simulink model "DoorSystem_Test"  (R2019b)
settings: Solver=ode1  StartTime=0.0  StopTime=inf  FixedStep=0.05  RelTol=1e-3  EnableMultiTasking=on
PostLoadFcn:
  | set_up_test_model
undefined symbols (not defined in the file): Enabled, MaxVehicles, Orientation, Z_DoorSystemPrm
libraries: TestBenchLib x22
settings Model: EnablePacing=on  OrderedModelArguments=off  Creator=godoyb  LastModifiedBy=bnadpurohit
settings DataIOCC: LimitDataPoints=on  ReturnWorkspaceOutputs=off
settings OptimizationCC: DefaultParameterBehavior=Inlined  LifeSpan=inf
settings DebuggingCC: FrameProcessingCompatibilityMsg=warning  AllowSymbolicDim=off  SFUnexpectedBacktrackingDiag=warning  SFNoUnconditionalDefaultTransitionDiag=warning  SFExecutionAtInitializationDiag=none  ArithmeticOperatorsInVariantConditions=warning
settings HardwareCC: ProdBitPerPointer=32  ProdBitPerSizeT=32  ProdBitPerPtrDiffT=32  ProdLargestAtomicFloat=None  ProdIntDivRoundTo=Undefined  ProdEndianess=Unspecified  ProdWordSize=32  ProdHWDeviceType=Custom Processor->Custom
settings ModelReferenceCC: PropagateSignalLabelsOutOfModel=off
settings SFSimCC: SimUseLocalCustomCode=off  CustomCodeUndefinedFunction=UseInterfaceOnly
settings RTWCC: RTWUseLocalCustomCode=off  TargetLang=C++
settings CodeAppCC: StateflowObjectComments=on
settings GRTTargetCC: TargetLangStandard=C++03 (ISO)  MultiInstanceERTCode=on  CodeInterfacePackaging=C++ class
settings ConfigComp: CovMetricSettings=dw  CovHtmlReporting=on  CovSaveCumulativeToWorkspaceVar=on  CovSaveSingleToWorkspaceVar=on  CovExternalEMLEnable=off

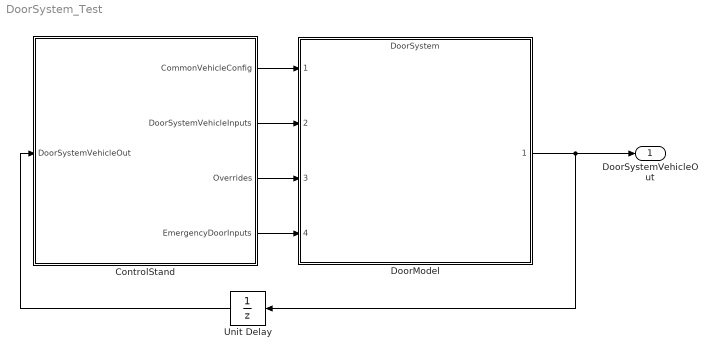
== system DoorSystem_Test ==
  ControlStand : Subsystem
  DoorModel : ModelReference  ModelNameDialog=DoorSystem.slx  ParameterArgumentNames=PRM_DoorSystem  ParameterArgumentValues=[Z_DoorSystemPrm]  UsingDefaultArgumentValue=0  SimulationMode=Normal  ModelReferenceVersion=1.2191
  Unit Delay : UnitDelay  SampleTime=-1  HasFrameUpgradeWarning=on
  DoorSystemVehicleOut : Outport  VectorParamsAs1DForOutWhenUnconnected=off
  wires:
  DoorModel/1 -> Unit Delay/1, DoorSystemVehicleOut/1
  ControlStand/1(CommonVehicleConfig) -> DoorModel/1
  ControlStand/2(DoorSystemVehicleInputs) -> DoorModel/2
  ControlStand/3(Overrides) -> DoorModel/3
  Unit Delay/1 -> ControlStand/1(DoorSystemVehicleOut)
  ControlStand/4(EmergencyDoorInputs) -> DoorModel/4

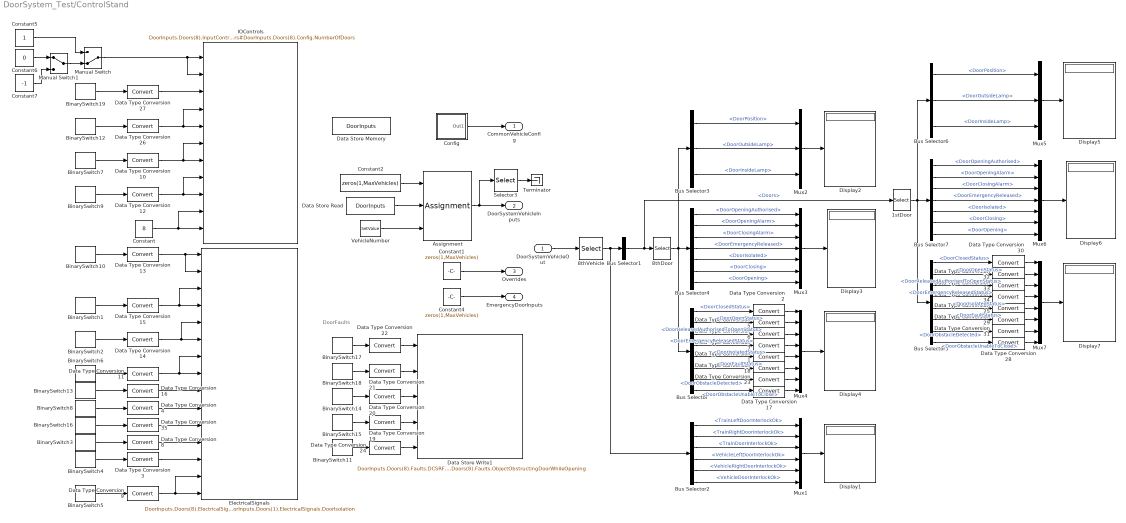
== system DoorSystem_Test/ControlStand ==
  note: DoorFaults
  DoorSystemVehicleOut : Inport
  1stDoor : Selector  InputPortWidth=16  IndexOptions=Index vector (dialog)  Indices=1  OutputSizes=1
  8thDoor : Selector  InputPortWidth=16  IndexOptions=Index vector (dialog)  Indices=16  OutputSizes=1
  8thVehicle : Selector  InputPortWidth=MaxVehicles  IndexOptions=Index vector (dialog)  Indices=8  OutputSizes=1
  Assignment : Assignment  DiagnosticForDimensions=Warning  IndexOptions=Index vector (port)  Indices=1  OutputSizes=1
  BinarySwitch{1..2,6,10} (4 alike) : TestBenchLib/BinarySwitch  value=1  init_value=1  block_colour=[0 1 0]  WorkspaceVarName=0
      settings: SourceProductName=Sydac Utilities
  BinarySwitch{3..5,7..9,11..19} (15 alike) : TestBenchLib/BinarySwitch  value=0  init_value=0  block_colour=[0 1 0]  WorkspaceVarName=0
      settings: SourceProductName=Sydac Utilities
  Bus Selector : BusSelector  OutputSignals=TCMS.DoorClosedStatus,TCMS.DoorOpenStatus,TCMS.DoorReleasedAuthorisedToOpenStatus,TCMS.DoorEmergencyReleasedStatus,TCMS.DoorIsolatedStatus,TCMS.DoorFaultStatus,TCMS.DoorObstacleDetected,TCMS.DoorObstacleUnableToClose
  Bus Selector1 : BusSelector  OutputSignals=Doors
  Bus Selector2 : BusSelector  OutputSignals=VehicleElectrical.TrainLeftDoorInterlockOk,VehicleElectrical.TrainRightDoorInterlockOk,VehicleElectrical.TrainDoorInterlockOk,VehicleElectrical.VehicleLeftDoorInterlockOk,VehicleElectrical.VehicleRightDoorInterlockOk,VehicleElectrical.VehicleDoorInterlockOk
  Bus Selector3 : BusSelector  OutputSignals=OutputControlStates.DoorPosition,OutputControlStates.DoorOutsideLamp,OutputControlStates.DoorInsideLamp
  Bus Selector4 : BusSelector  OutputSignals=Audio.DoorOpeningAuthorised,Audio.DoorOpeningAlarm,Audio.DoorClosingAlarm,Audio.DoorEmergencyReleased,Audio.DoorIsolated,Audio.DoorClosing,Audio.DoorOpening
  Bus Selector5 : BusSelector  OutputSignals=TCMS.DoorClosedStatus,TCMS.DoorOpenStatus,TCMS.DoorReleasedAuthorisedToOpenStatus,TCMS.DoorEmergencyReleasedStatus,TCMS.DoorIsolatedStatus,TCMS.DoorFaultStatus,TCMS.DoorObstacleDetected,TCMS.DoorObstacleUnableToClose
  Bus Selector6 : BusSelector  OutputSignals=OutputControlStates.DoorPosition,OutputControlStates.DoorOutsideLamp,OutputControlStates.DoorInsideLamp
  Bus Selector7 : BusSelector  OutputSignals=Audio.DoorOpeningAuthorised,Audio.DoorOpeningAlarm,Audio.DoorClosingAlarm,Audio.DoorEmergencyReleased,Audio.DoorIsolated,Audio.DoorClosing,Audio.DoorOpening
  Config : Subsystem
  Constant : Constant  Value=8
  Constant1 : Constant  Value=zeros(1,MaxVehicles)  OutDataTypeStr=Bus: BD_DoorSystem_In_Overrides
  Constant2 : Constant  Value=zeros(1,MaxVehicles)  OutDataTypeStr=Bus: BD_DoorSystem_In_Vehicle
  Constant4 : Constant  Value=zeros(1,MaxVehicles)  OutDataTypeStr=Bus: BD_DoorSystem_In_Emergency_Door
  Constant5 : Constant
  Constant6 : Constant  Value=0
  Constant7 : Constant  Value=-1
  Data Store Memory : DataStoreMemory  DataStoreName=DoorInputs  ReadBeforeWriteMsg=warning  WriteAfterWriteMsg=warning  WriteAfterReadMsg=warning  ShowAdditionalParam=off  OutDataTypeStr=Bus: BD_DoorSystem_In_Vehicle
  Data Store Read : DataStoreRead  DataStoreName=DoorInputs
  Data Store Write1 : DataStoreWrite  DataStoreName=DoorInputs  DataStoreElements=DoorInputs.Doors(8).Faults.DCSRFailure#DoorInputs.Doors(8).Faults.DoorUnauthorisedOpen#DoorInputs.Doors(1).Faults.DCSRFailure#DoorInputs.Doors(8).Faults.ObjectObstructingDoorWhileClosing#DoorInputs.Doors(8).Faults.ObjectObstructingDoorWhileOpening
  Data Type Conversion{1..35} (35 alike) : DataTypeConversion
  Display{1..7} (7 alike) : Display
  ElectricalSignals : DataStoreWrite  DataStoreName=DoorInputs  DataStoreElements=DoorInputs.Doors(8).ElectricalSignals.DoorControlPower#DoorInputs.Doors(1).ElectricalSignals.DoorControlPower#DoorInputs.Doors(8).ElectricalSignals.DoorMotorPower#DoorInputs.Doors(1).ElectricalSignals.DoorMotorPower#DoorInputs.Doors(8).ElectricalSignals.DoorEnable#DoorInputs.Doors(1).ElectricalSignals.DoorEnable#DoorInputs.Doors(8).ElectricalSignals.DoorRelease#DoorInputs.Doors(1).ElectricalSignals.DoorRelease#DoorInputs.Doors(8).ElectricalSignals.DoorOpen#DoorInputs.Doors(1).ElectricalSignals.DoorOpen#DoorInputs.Doors(8).ElectricalSignals.DoorClose#DoorInputs.Doors(1).ElectricalSignals.DoorClose#DoorInputs.Doors(8).ElectricalSignals.DoorEmergencyRelease#DoorInputs.Doors(8).ElectricalSignals.DoorIsolation#DoorInputs.Doors(1).ElectricalSignals.DoorIsolation
  IOControls : DataStoreWrite  DataStoreName=DoorInputs  DataStoreElements=DoorInputs.Doors(8).InputControlStates.OpenCloseWidget#DoorInputs.Doors(1).InputControlStates.OpenCloseWidget#DoorInputs.Doors(8).InputControlStates.LocalDoorOpenPB#DoorInputs.Doors(8).InputControlStates.EmergencyAccessDevice#DoorInputs.Doors(1).InputControlStates.EmergencyAccessDevice#DoorInputs.Doors(8).InputControlStates.EmergencyEgressDevice#DoorInputs.Doors(1).InputControlStates.EmergencyEgressDevice#DoorInputs.Doors(8).InputControlStates.LocalDoorIsolationLock#DoorInputs.Doors(1).InputControlStates.LocalDoorIsolationLock#DoorInputs.Doors(1).Config.NumberOfDoors#DoorInputs.Doors(8).Config.NumberOfDoors
  Manual Switch : ManualSwitch  CurrentSetting=0
  Manual Switch1 : ManualSwitch
  Mux1 : Mux  Inputs=6
  Mux2 : Mux  Inputs=3
  Mux3 : Mux  Inputs=7
  Mux4 : Mux  Inputs=8
  Mux5 : Mux  Inputs=3
  Mux6 : Mux  Inputs=7
  Mux7 : Mux  Inputs=8
  Selector3 : Selector  InputPortWidth=MaxVehicles  IndexOptions=Index vector (dialog)  Indices=8  OutputSizes=1
  Terminator : Terminator
  VehicleNumber : TestBenchLib/SetValue  value=8  init_value=8  WorkspaceVarName=0
      settings: SourceProductName=Sydac Utilities
  CommonVehicleConfig : Outport  VectorParamsAs1DForOutWhenUnconnected=off
  DoorSystemVehicleInputs : Outport  Port=2  VectorParamsAs1DForOutWhenUnconnected=off
  Overrides : Outport  Port=3  VectorParamsAs1DForOutWhenUnconnected=off
  EmergencyDoorInputs : Outport  Port=4
  wires:
  Constant1/1 -> Overrides/1
  Config/1(Out1) -> CommonVehicleConfig/1
  Assignment/1 -> DoorSystemVehicleInputs/1, Selector3/1
  Bus Selector1/1 -> 1stDoor/1, 8thDoor/1  "<Doors>"
  Mux4/1 -> Display4/1
  8thVehicle/1 -> Bus Selector1/1, Bus Selector2/1
  Bus Selector/1 -> Data Type Conversion2/1  "<DoorClosedStatus>"
  DoorSystemVehicleOut/1 -> 8thVehicle/1
  BinarySwitch1/1 -> Data Type Conversion15/1
  Bus Selector2/1 -> Mux1/1  "<TrainLeftDoorInterlockOk>"
  Bus Selector2/2 -> Mux1/2  "<TrainRightDoorInterlockOk>"
  Bus Selector2/4 -> Mux1/4  "<VehicleLeftDoorInterlockOk>"
  Bus Selector2/5 -> Mux1/5  "<VehicleRightDoorInterlockOk>"
  Mux1/1 -> Display1/1
  Bus Selector/2 -> Data Type Conversion5/1  "<DoorOpenStatus>"
  Bus Selector/3 -> Data Type Conversion6/1  "<DoorReleasedAuthorisedToOpenStatus>"
  Data Type Conversion2/1 -> Mux4/1
  Data Type Conversion5/1 -> Mux4/2
  Data Type Conversion6/1 -> Mux4/3
  Data Type Conversion7/1 -> Mux4/4
  8thDoor/1 -> Bus Selector3/1, Bus Selector/1, Bus Selector4/1
  Bus Selector3/1 -> Mux2/1  "<DoorPosition>"
  Bus Selector3/3 -> Mux2/3  "<DoorInsideLamp>"
  Mux3/1 -> Display3/1
  BinarySwitch15/1 -> Data Type Conversion19/1
  BinarySwitch14/1 -> Data Type Conversion20/1
  BinarySwitch17/1 -> Data Type Conversion22/1
  BinarySwitch18/1 -> Data Type Conversion21/1
  Data Type Conversion27/1 -> IOControls/3
  BinarySwitch19/1 -> Data Type Conversion27/1
  Data Type Conversion19/1 -> Data Store Write1/4
  Data Type Conversion20/1 -> Data Store Write1/3
  Data Type Conversion21/1 -> Data Store Write1/2
  Data Type Conversion22/1 -> Data Store Write1/1
  Bus Selector2/3 -> Mux1/3  "<TrainDoorInterlockOk>"
  Bus Selector2/6 -> Mux1/6  "<VehicleDoorInterlockOk>"
  Data Type Conversion1/1 -> Mux4/5
  Mux2/1 -> Display2/1
  Bus Selector4/1 -> Mux3/1  "<DoorOpeningAuthorised>"
  Bus Selector4/2 -> Mux3/2  "<DoorOpeningAlarm>"
  Bus Selector4/3 -> Mux3/3  "<DoorClosingAlarm>"
  Bus Selector4/4 -> Mux3/4  "<DoorEmergencyReleased>"
  Bus Selector4/5 -> Mux3/5  "<DoorIsolated>"
  Bus Selector4/6 -> Mux3/6  "<DoorClosing>"
  Bus Selector4/7 -> Mux3/7  "<DoorOpening>"
  BinarySwitch7/1 -> Data Type Conversion10/1
  Data Type Conversion12/1 -> IOControls/8, IOControls/9
  BinarySwitch9/1 -> Data Type Conversion12/1
  Data Type Conversion13/1 -> ElectricalSignals/2, ElectricalSignals/1
  BinarySwitch10/1 -> Data Type Conversion13/1
  Data Type Conversion18/1 -> Mux4/6
  Data Type Conversion23/1 -> Mux4/7
  Data Type Conversion17/1 -> Mux4/8
  Bus Selector/4 -> Data Type Conversion7/1  "<DoorEmergencyReleasedStatus>"
  Bus Selector/5 -> Data Type Conversion1/1  "<DoorIsolatedStatus>"
  Bus Selector/6 -> Data Type Conversion18/1  "<DoorFaultStatus>"
  Bus Selector/7 -> Data Type Conversion23/1  "<DoorObstacleDetected>"
  Bus Selector/8 -> Data Type Conversion17/1  "<DoorObstacleUnableToClose>"
  Bus Selector3/2 -> Mux2/2  "<DoorOutsideLamp>"
  BinarySwitch11/1 -> Data Type Conversion24/1
  Data Type Conversion24/1 -> Data Store Write1/5
  Bus Selector6/2 -> Mux5/2  "<DoorOutsideLamp>"
  Bus Selector5/8 -> Data Type Conversion28/1  "<DoorObstacleUnableToClose>"
  1stDoor/1 -> Bus Selector6/1, Bus Selector5/1, Bus Selector7/1
  Bus Selector7/2 -> Mux6/2  "<DoorOpeningAlarm>"
  Bus Selector7/1 -> Mux6/1  "<DoorOpeningAuthorised>"
  Bus Selector5/4 -> Data Type Conversion34/1  "<DoorEmergencyReleasedStatus>"
  Data Type Conversion31/1 -> Mux7/7
  Data Type Conversion34/1 -> Mux7/4
  Data Type Conversion25/1 -> Mux7/5
  Data Type Conversion29/1 -> Mux7/6
  Bus Selector7/7 -> Mux6/7  "<DoorOpening>"
  Bus Selector7/6 -> Mux6/6  "<DoorClosing>"
  Mux6/1 -> Display6/1
  Bus Selector5/6 -> Data Type Conversion29/1  "<DoorFaultStatus>"
  Bus Selector7/4 -> Mux6/4  "<DoorEmergencyReleased>"
  Bus Selector7/5 -> Mux6/5  "<DoorIsolated>"
  Bus Selector7/3 -> Mux6/3  "<DoorClosingAlarm>"
  Mux5/1 -> Display5/1
  Mux7/1 -> Display7/1
  Data Type Conversion28/1 -> Mux7/8
  Bus Selector5/2 -> Data Type Conversion32/1  "<DoorOpenStatus>"
  Data Type Conversion33/1 -> Mux7/3
  Bus Selector5/7 -> Data Type Conversion31/1  "<DoorObstacleDetected>"
  Bus Selector5/5 -> Data Type Conversion25/1  "<DoorIsolatedStatus>"
  Bus Selector5/3 -> Data Type Conversion33/1  "<DoorReleasedAuthorisedToOpenStatus>"
  Data Type Conversion32/1 -> Mux7/2
  Bus Selector6/3 -> Mux5/3  "<DoorInsideLamp>"
  Bus Selector5/1 -> Data Type Conversion30/1  "<DoorClosedStatus>"
  Data Type Conversion30/1 -> Mux7/1
  Bus Selector6/1 -> Mux5/1  "<DoorPosition>"
  Selector3/1 -> Terminator/1
  Data Store Read/1 -> Assignment/2
  VehicleNumber/1 -> Assignment/3
  Constant2/1 -> Assignment/1
  Constant4/1 -> EmergencyDoorInputs/1
  BinarySwitch2/1 -> Data Type Conversion14/1
  BinarySwitch8/1 -> Data Type Conversion4/1
  BinarySwitch3/1 -> Data Type Conversion8/1
  BinarySwitch5/1 -> Data Type Conversion9/1
  BinarySwitch4/1 -> Data Type Conversion3/1
  Constant/1 -> IOControls/11, IOControls/10
  Data Type Conversion10/1 -> IOControls/6, IOControls/7
  Data Type Conversion26/1 -> IOControls/4, IOControls/5
  BinarySwitch12/1 -> Data Type Conversion26/1
  Data Type Conversion3/1 -> ElectricalSignals/13
  Data Type Conversion9/1 -> ElectricalSignals/14, ElectricalSignals/15
  Data Type Conversion8/1 -> ElectricalSignals/12
  Data Type Conversion4/1 -> ElectricalSignals/10
  Data Type Conversion15/1 -> ElectricalSignals/3, ElectricalSignals/4
  BinarySwitch6/1 -> Data Type Conversion11/1
  Data Type Conversion11/1 -> ElectricalSignals/7, ElectricalSignals/8
  Data Type Conversion14/1 -> ElectricalSignals/5, ElectricalSignals/6
  Manual Switch1/1 -> Manual Switch/2
  Constant5/1 -> Manual Switch/1
  Constant6/1 -> Manual Switch1/1
  Constant7/1 -> Manual Switch1/2
  Manual Switch/1 -> IOControls/2, IOControls/1
  Data Type Conversion16/1 -> ElectricalSignals/9
  BinarySwitch13/1 -> Data Type Conversion16/1
  Data Type Conversion35/1 -> ElectricalSignals/11
  BinarySwitch16/1 -> Data Type Conversion35/1

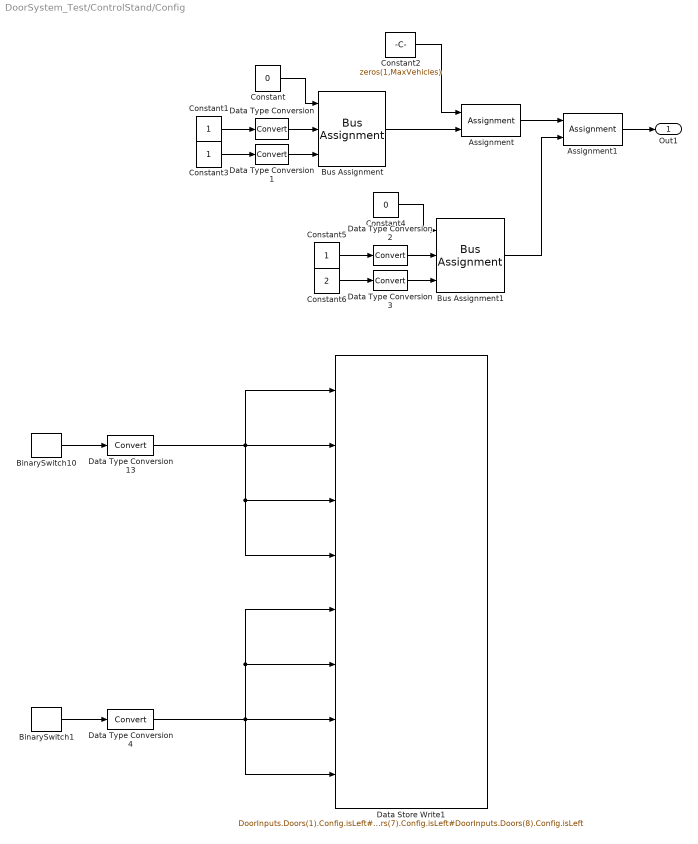
== system DoorSystem_Test/ControlStand/Config ==
  Assignment : Assignment  DiagnosticForDimensions=Warning  IndexOptions=Index vector (dialog)  Indices=[1,2,3,4]  OutputSizes=1
  Assignment1 : Assignment  DiagnosticForDimensions=Warning  IndexOptions=Index vector (dialog)  Indices=[5,6,7,8]  OutputSizes=1
  BinarySwitch1 : TestBenchLib/BinarySwitch  value=0  init_value=0  block_colour=[0 1 0]  WorkspaceVarName=0
      settings: SourceProductName=Sydac Utilities
  BinarySwitch10 : TestBenchLib/BinarySwitch  value=1  init_value=1  block_colour=[0 1 0]  WorkspaceVarName=0
      settings: SourceProductName=Sydac Utilities
  Bus Assignment : BusAssignment  AssignedSignals=Enabled,Orientation
  Bus Assignment1 : BusAssignment  AssignedSignals=Enabled,Orientation
  Constant : Constant  Value=0  OutDataTypeStr=Bus: BD_CommonTrain_Cfg_Vehicle
  Constant1 : Constant
  Constant2 : Constant  Value=zeros(1,MaxVehicles)  OutDataTypeStr=Bus: BD_CommonTrain_Cfg_Vehicle
  Constant3 : Constant
  Constant4 : Constant  Value=0  OutDataTypeStr=Bus: BD_CommonTrain_Cfg_Vehicle
  Constant5 : Constant
  Constant6 : Constant  Value=2
  Data Store Write1 : DataStoreWrite  DataStoreName=DoorInputs  DataStoreElements=DoorInputs.Doors(1).Config.isLeft#DoorInputs.Doors(2).Config.isLeft#DoorInputs.Doors(3).Config.isLeft#DoorInputs.Doors(4).Config.isLeft#DoorInputs.Doors(5).Config.isLeft#DoorInputs.Doors(6).Config.isLeft#DoorInputs.Doors(7).Config.isLeft#DoorInputs.Doors(8).Config.isLeft
  Data Type Conversion{,1..4,13} (6 alike) : DataTypeConversion
  Out1 : Outport  VectorParamsAs1DForOutWhenUnconnected=off
  wires:
  Assignment/1 -> Assignment1/1
  Constant/1 -> Bus Assignment/1
  Constant1/1 -> Data Type Conversion/1
  Constant2/1 -> Assignment/1
  Bus Assignment/1 -> Assignment/2
  Data Type Conversion/1 -> Bus Assignment/2
  Assignment1/1 -> Out1/1
  Constant3/1 -> Data Type Conversion1/1
  Data Type Conversion1/1 -> Bus Assignment/3
  Data Type Conversion3/1 -> Bus Assignment1/3
  Constant6/1 -> Data Type Conversion3/1
  Data Type Conversion2/1 -> Bus Assignment1/2
  Constant5/1 -> Data Type Conversion2/1
  Constant4/1 -> Bus Assignment1/1
  Bus Assignment1/1 -> Assignment1/2
  BinarySwitch10/1 -> Data Type Conversion13/1
  BinarySwitch1/1 -> Data Type Conversion4/1
  Data Type Conversion13/1 -> Data Store Write1/2, Data Store Write1/3, Data Store Write1/4, Data Store Write1/1
  Data Type Conversion4/1 -> Data Store Write1/8, Data Store Write1/7, Data Store Write1/6, Data Store Write1/5
